simulink model "examen_simulacion_16_12_22"  (R2024a)
settings: Solver=VariableStepAuto  StartTime=0.0  StopTime=10  FixedStep=0.006  MaxStep=0.1  RelTol=1e-3
values from neighbouring files (symbols this model uses):
  A = (2-(a_adelanto*h_digitalizacion))/(2+(a_adelanto*h_digitalizacion))    [examen_16_12_22.m]
  a_adelanto = y + Pd1_real    [examen_16_12_22.m]
  B = K_rlocfind*(2+(b_adelanto*h_digitalizacion))/(2+(a_adelanto*h_digitalizacion))    [examen_16_12_22.m]
  b_adelanto = Pd1_real    [examen_16_12_22.m]
  C = K_rlocfind*((b_adelanto*h_digitalizacion)-2)/(2+(a_adelanto*h_digitalizacion))    [examen_16_12_22.m]
  G_den = den    [examen_16_12_22.m]
  G_num = num    [examen_16_12_22.m]
  h_digitalizacion = 0.006    [examen_16_12_22.m]
undefined symbols (not defined in the file or in its folder): K_rlocfind
libraries: simulink x1
settings Model: Creator=david  LastModifiedBy=david

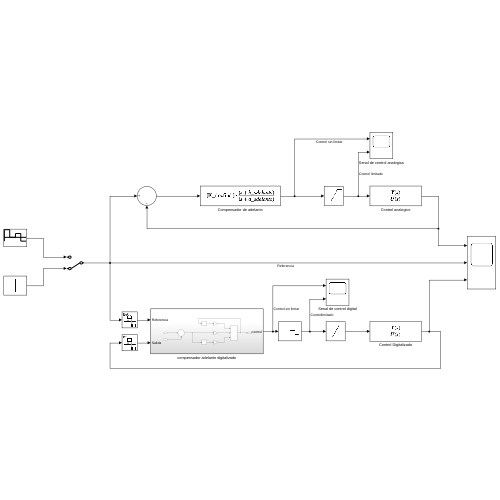
[thumbnail: Simulink's stored preview of the top-level diagram]
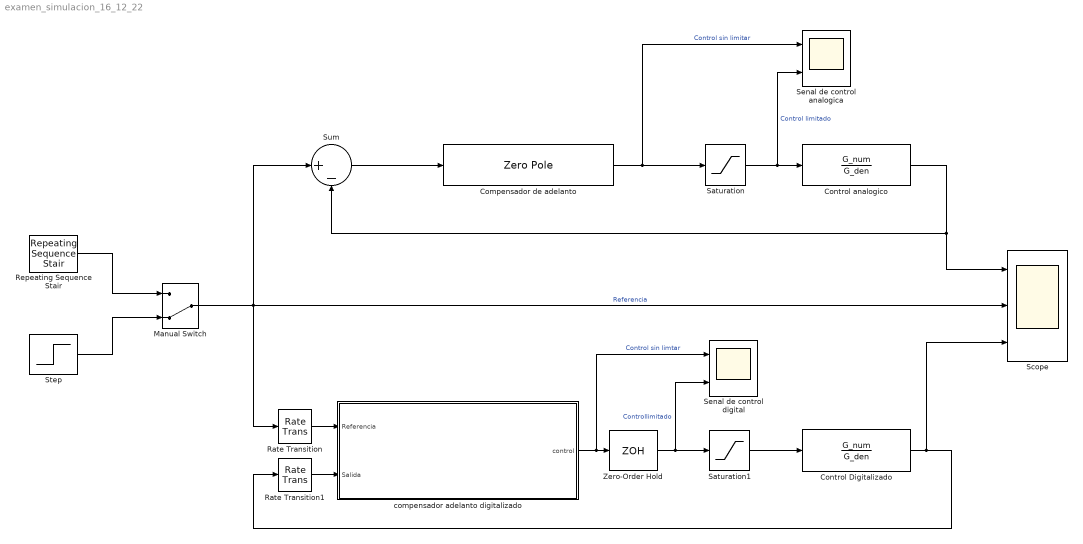
== system examen_simulacion_16_12_22 ==
  Compensador de adelanto : ZeroPole  Zeros=[-b_adelanto]  Poles=[-a_adelanto]  Gain=[K_rlocfind]
  Control Digitalizado : TransferFcn  Numerator=G_num  Denominator=G_den
  Control analogico : TransferFcn  Numerator=G_num  Denominator=G_den
  Manual Switch : ManualSwitch  CurrentSetting=0
  Rate Transition : RateTransition  Integrity=off  OutPortSampleTime=h_digitalizacion
  Rate Transition1 : RateTransition  Integrity=off  OutPortSampleTime=h_digitalizacion
  Repeating Sequence Stair : simulink/Sources/Repeating Sequence Stair  OutValues=[2 0 1 -1].'  tsamp=4  OutMin=[]  OutMax=[]  OutDataTypeStr=double  OutputDataTypeScalingMode=double  OutDataType=fixdt(0,8)  ConRadixGroup=Best Precision: Vector-wise  OutScaling=2^-12
  Saturation : Saturate  UpperLimit=9  LowerLimit=-9
  Saturation1 : Saturate  UpperLimit=9  LowerLimit=-9
  Scope : Scope  NumInputPorts=3
  Senal de control analogica : Scope  NumInputPorts=2
  Senal de control digital : Scope  NumInputPorts=2
  Step : Step  SampleTime=h_digitalizacion
  Sum : Sum  Inputs=|+-
  Zero-Order Hold : ZeroOrderHold  SampleTime=h_digitalizacion
  compensador adelanto digitalizado : Subsystem
  wires:
  Compensador de adelanto/1 -> Saturation/1, Senal de control analogica/1  "Control sin limitar"
  Saturation/1 -> Control analogico/1, Senal de control analogica/2  "Control limitado"
  Control analogico/1 -> Sum/2, Scope/1
  Sum/1 -> Compensador de adelanto/1
  Step/1 -> Manual Switch/2
  Repeating Sequence Stair/1 -> Manual Switch/1
  Manual Switch/1 -> Sum/1, Rate Transition/1, Scope/2  "Referencia"
  Saturation1/1 -> Control Digitalizado/1
  Control Digitalizado/1 -> Rate Transition1/1, Scope/3
  compensador adelanto digitalizado/1(control) -> Senal de control digital/1, Zero-Order Hold/1  "Control sin limtar"
  Rate Transition1/1 -> compensador adelanto digitalizado/2(Salida)
  Rate Transition/1 -> compensador adelanto digitalizado/1(Referencia)
  Zero-Order Hold/1 -> Senal de control digital/2, Saturation1/1  "Controllimitado"

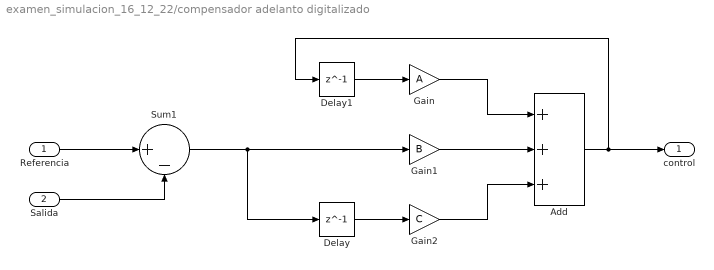
== system examen_simulacion_16_12_22/compensador adelanto digitalizado ==
  Referencia : Inport
  Salida : Inport  Port=2
  Add : Sum  Inputs=+++
  Delay : Delay  DelayLength=1  SampleTime=h_digitalizacion
  Delay1 : Delay  DelayLength=1  SampleTime=h_digitalizacion
  Gain : Gain  Gain=A
  Gain1 : Gain  Gain=B
  Gain2 : Gain  Gain=C
  Sum1 : Sum  Inputs=|+-
  control : Outport
  wires:
  Add/1 -> control/1, Delay1/1
  Gain1/1 -> Add/2
  Sum1/1 -> Delay/1, Gain1/1
  Delay/1 -> Gain2/1
  Delay1/1 -> Gain/1
  Salida/1 -> Sum1/2
  Gain/1 -> Add/1
  Gain2/1 -> Add/3
  Referencia/1 -> Sum1/1
